simulink subsystem "s0312_simulator"  (R2021a)
settings: Solver=VariableStepAuto  StartTime=0.0  StopTime=10.0  RelTol=1e-3
model mask{th_0=0, th_dot_0=0, al_0=0, al_dot_0=0}
  mask prompts: th_0 "Initial theta"; th_dot_0 "Initial theta dot"; al_0 "Initial alpha"; al_dot_0 "Initial aplha dot"
settings Model: Creator=paolo  LastModifiedBy=paolo

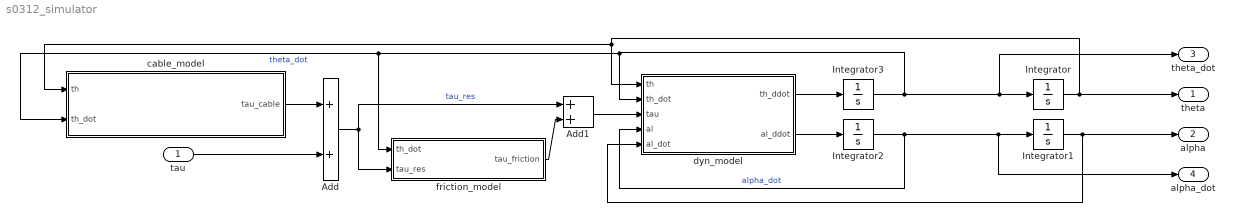
== system s0312_simulator ==
  tau : Inport  Unit=N*m  PortDimensions=1
  Add : Sum
  Add1 : Sum
  Integrator : Integrator  InitialCondition=th_0  LimitOutput=on  UpperSaturationLimit=135 * pi / 180  LowerSaturationLimit=- 135 * pi / 180
  Integrator1 : Integrator  InitialCondition=al_0  UpperSaturationLimit=0.01  LowerSaturationLimit=-0.01  WrapState=on
  Integrator2 : Integrator  InitialCondition=al_dot_0  UpperSaturationLimit=0.01  LowerSaturationLimit=-0.01
  Integrator3 : Integrator  InitialCondition=th_dot_0  UpperSaturationLimit=90  LowerSaturationLimit=-90
  cable_model : MATLAB Function  TreatAsAtomicUnit=on
  dyn_model : MATLAB Function  TreatAsAtomicUnit=on
  friction_model : MATLAB Function  TreatAsAtomicUnit=on
  theta : Outport  Unit=rad  PortDimensions=1
  alpha : Outport  Port=2  PortDimensions=1
  theta_dot : Outport  Port=3  Unit=rad/s  PortDimensions=1
  alpha_dot : Outport  Port=4  PortDimensions=1
  wires:
  dyn_model/1(th_ddot) -> Integrator3/1
  Integrator/1 -> dyn_model/1(th), cable_model/1(th), theta/1
  Integrator2/1 -> dyn_model/4(al), Integrator1/1, alpha_dot/1  "alpha_dot"
  Integrator3/1 -> cable_model/2(th_dot), friction_model/1(th_dot), dyn_model/2(th_dot), Integrator/1, theta_dot/1  "theta_dot"
  dyn_model/2(al_ddot) -> Integrator2/1
  Integrator1/1 -> alpha/1, dyn_model/5(al_dot)
  tau/1 -> Add/2
  cable_model/1(tau_cable) -> Add/1
  Add1/1 -> dyn_model/3(tau)
  Add/1 -> friction_model/2(tau_res), Add1/1  "tau_res"
  friction_model/1(tau_friction) -> Add1/2

== matlab function s0312_simulator/cable_model ==
  data: th input; th_dot input; tau_cable output
function tau_cable = cable_model(th,th_dot)
%#codegen

%    This function was generated by the Symbolic Math Toolbox version 8.7.
%    13-Mar-2022 23:50:13

tau_cable = th.*(-1.432394487827058e-3)-pi.*2.431091755728701e-4;

== matlab function s0312_simulator/dyn_model ==
  data: th input; th_dot input size=1; tau input size=1; th_ddot output; al input size=1; al_dot input size=1; al_ddot output size=1
function [th_ddot,al_ddot] = dyn_model(th,th_dot,tau,al,al_dot)
%#codegen

%    This function was generated by the Symbolic Math Toolbox version 8.7.
%    13-Mar-2022 23:50:13

t2 = cos(al);
t3 = sin(al);
t4 = al.*2.0;
t5 = al_dot.^2;
t6 = th_dot.^2;
t7 = t2.^2;
t8 = sin(t4);
t9 = t3.^3;
t10 = t7.*6.89688e+5;
t11 = t10-1.506113e+6;
t12 = 1.0./t11;
th_ddot = t12.*(t8.*1.1256975e+7+tau.*1.5e+9-th_dot.*3.33555e+5+al_dot.*t2.*2.099747093023256e+4+t3.*t5.*1.9737e+5-t6.*(t3-t9).*1.480275e+5-al_dot.*t8.*th_dot.*1.49769e+5).*-2.0;
if nargout > 1
    et1 = al_dot.*1.60229842099333e+5+t3.*1.376337296511628e+8+t9.*3.416823e+7-al_dot.*t7.*3.186675e+4+t5.*t8.*1.95075e+5-t6.*t8.*5.64792375e+5+t2.*tau.*2.965116279069767e+9;
    et2 = t2.*th_dot.*(-6.593529069767442e+5)+t2.^3.*t3.*t6.*2.246535e+5-al_dot.*t3.*th_dot.*5.9211e+5+al_dot.*t9.*th_dot.*5.9211e+5;
    al_ddot = t12.*(et1+et2);
end

== matlab function s0312_simulator/friction_model ==
  data: th_dot input; tau_friction output; tau_res input
function tau_friction = friction_model(th_dot,tau_res)
%#codegen

%    This function was generated by the Symbolic Math Toolbox version 8.7.
%    13-Mar-2022 23:50:13

if ((-1.0e-8 < th_dot) & (th_dot < 1.0e-8))
    tau_friction = min([1.2e-3,tau_res]);
else
    tau_friction = sign(th_dot).*1.24e-3+min([0.0,tau_res]);
end
